simulink model "Linear_Model"  (R2018a)
settings: Solver=VariableStepAuto  StartTime=0.0  StopTime=300  RelTol=1e-3
values from neighbouring files (symbols this model uses):
  A_lat = [a11_lat, a12_lat, a13_lat, a14_lat, a15_lat ... (first row only)    [cont_code-1.m]    (also in flight_controller.m)
  A_long = [a11_long, a12_long, a13_long, a14_long, a15_long ... (first row only)    [cont_code-1.m]    (also in flight_controller.m)
  B_lat = [b11_lat, b12_lat ... (first row only)    [cont_code-1.m]    (also in flight_controller.m)
  B_long = [b11_long, b12_long ... (first row only)    [cont_code-1.m]    (also in flight_controller.m)
  C_lat = eye(5)    [cont_code-1.m]    (also in flight_controller.m)
  C_long = eye(5)    [cont_code-1.m]    (also in flight_controller.m)
  D_lat = zeros(5,2)    [cont_code-1.m]    (also in flight_controller.m)
  D_long = [0, 0 ... (first row only)    [cont_code-1.m]    (also in flight_controller.m)
libraries: simulink x2
settings Model: Creator=Navneet  LastModifiedBy=Sam
settings DebuggingCC: LibraryContextMissingDiagnostic=warning
settings SFSimCC: SimUseLocalCustomCode=on
settings RTWCC: RTWUseLocalCustomCode=on

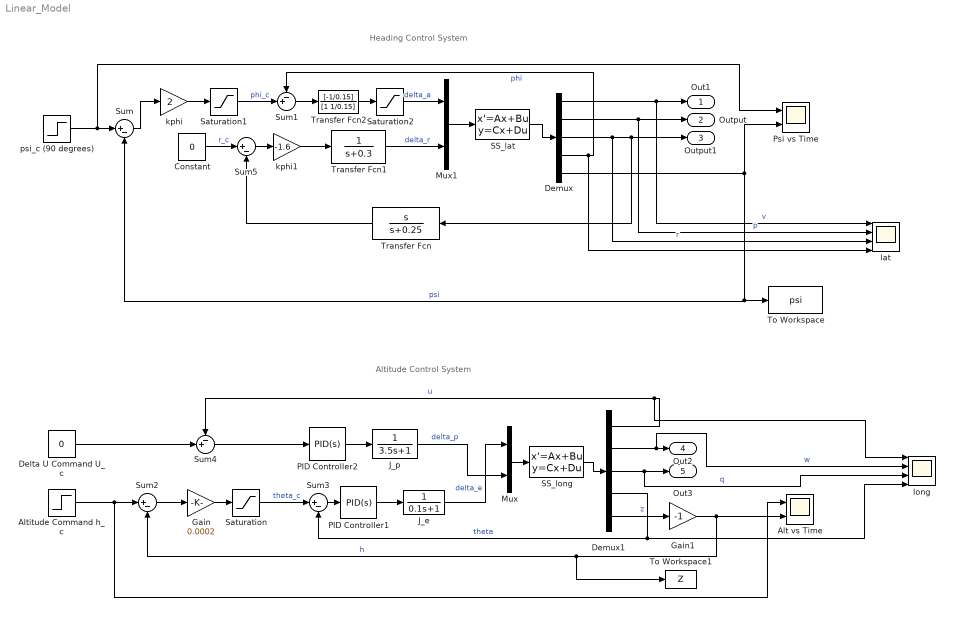
== system Linear_Model ==
  note: Altitude Control System
  note: Heading Control System
  Alt vs Time : Scope  NumInputPorts=2
  Altitude Command h_c : Step  After=1524  SampleTime=0
  Constant : Constant  Value=0
  Delta U Command U_c : Constant  Value=0
  Demux : Demux  Outputs=5
  Demux1 : Demux  Outputs=5
  Gain : Gain  Gain=0.0002
  Gain1 : Gain  Gain=-1
  J_e : TransferFcn  Denominator=[0.1 1]
  J_p : TransferFcn  Denominator=[3.5 1]
  Mux : Mux  Inputs=2
  Mux1 : Mux  Inputs=2
  PID Controller1 : simulink/Continuous/PID Controller  Controller=PID  TimeDomain=Continuous-time  SampleTime=-1  IntegratorMethod=Forward Euler  FilterMethod=Forward Euler  Form=Parallel  UseFilter=on  ControllerParametersSource=internal  P=-6.29147828725261  I=-1.81540038520091  D=-5.41857533868541  N=645.661916939529  InitialConditionSource=internal  InitialConditionForIntegrator=0  InitialConditionForFilter=0  ExternalReset=none  LimitOutput=off  UpperSaturationLimit=inf  LowerSaturationLimit=-inf  LinearizeAsGain=on  AntiWindupMode=none  Kb=1  TrackingMode=off  Kt=1  PParamMin=[]  PParamMax=[]  IParamMin=[]  IParamMax=[]  DParamMin=[]  DParamMax=[]  NParamMin=[]  NParamMax=[]  KbParamMin=[]  KbParamMax=[]  KtParamMin=[]  KtParamMax=[]  POutMin=[]  POutMax=[]  IOutMin=[]  IOutMax=[]  DOutMin=[]  DOutMax=[]  NOutMin=[]  NOutMax=[]  KbOutMin=[]  KbOutMax=[]  KtOutMin=[]  KtOutMax=[]  IntegratorOutMin=[]  IntegratorOutMax=[]  FilterOutMin=[]  FilterOutMax=[]  SumOutMin=[]  SumOutMax=[]  SumI1OutMin=[]  SumI1OutMax=[]  SumI2OutMin=[]  SumI2OutMax=[]  SumI3OutMin=[]  SumI3OutMax=[]  SumDOutMin=[]  SumDOutMax=[]  SaturationOutMin=[]  SaturationOutMax=[]  IntegratorContinuousStateAttributes=''  IntegratorStateMustResolveToSignalObject=off  IntegratorRTWStateStorageClass=Auto  FilterContinuousStateAttributes=''  FilterStateMustResolveToSignalObject=off  FilterRTWStateStorageClass=Auto  DifferentiatorICPrevScaledInput=0  DifferentiatorOutMin=[]  DifferentiatorOutMax=[]  FilterDiffOutCoefMin=[]  FilterDiffOutCoefMax=[]  SumDenOutMin=[]  SumDenOutMax=[]  SumNumOutMin=[]  SumNumOutMax=[]  ReciprocalOutMin=[]  ReciprocalOutMax=[]  DivideOutMin=[]  DivideOutMax=[]  TunerSelectOption=Transfer Function Based (PID Tuner App)
  PID Controller2 : simulink/Continuous/PID Controller  Controller=PID  TimeDomain=Continuous-time  SampleTime=-1  IntegratorMethod=Forward Euler  FilterMethod=Forward Euler  Form=Parallel  UseFilter=on  ControllerParametersSource=internal  P=23.4112253132064  I=10.8898679236466  D=12.4928821977603  N=1211.32658735594  InitialConditionSource=internal  InitialConditionForIntegrator=0  InitialConditionForFilter=0  ExternalReset=none  LimitOutput=off  UpperSaturationLimit=inf  LowerSaturationLimit=-inf  LinearizeAsGain=on  AntiWindupMode=none  Kb=1  TrackingMode=off  Kt=1  PParamMin=[]  PParamMax=[]  IParamMin=[]  IParamMax=[]  DParamMin=[]  DParamMax=[]  NParamMin=[]  NParamMax=[]  KbParamMin=[]  KbParamMax=[]  KtParamMin=[]  KtParamMax=[]  POutMin=[]  POutMax=[]  IOutMin=[]  IOutMax=[]  DOutMin=[]  DOutMax=[]  NOutMin=[]  NOutMax=[]  KbOutMin=[]  KbOutMax=[]  KtOutMin=[]  KtOutMax=[]  IntegratorOutMin=[]  IntegratorOutMax=[]  FilterOutMin=[]  FilterOutMax=[]  SumOutMin=[]  SumOutMax=[]  SumI1OutMin=[]  SumI1OutMax=[]  SumI2OutMin=[]  SumI2OutMax=[]  SumI3OutMin=[]  SumI3OutMax=[]  SumDOutMin=[]  SumDOutMax=[]  SaturationOutMin=[]  SaturationOutMax=[]  IntegratorContinuousStateAttributes=''  IntegratorStateMustResolveToSignalObject=off  IntegratorRTWStateStorageClass=Auto  FilterContinuousStateAttributes=''  FilterStateMustResolveToSignalObject=off  FilterRTWStateStorageClass=Auto  DifferentiatorICPrevScaledInput=0  DifferentiatorOutMin=[]  DifferentiatorOutMax=[]  FilterDiffOutCoefMin=[]  FilterDiffOutCoefMax=[]  SumDenOutMin=[]  SumDenOutMax=[]  SumNumOutMin=[]  SumNumOutMax=[]  ReciprocalOutMin=[]  ReciprocalOutMax=[]  DivideOutMin=[]  DivideOutMax=[]  TunerSelectOption=Transfer Function Based (PID Tuner App)
  Psi vs Time : Scope  NumInputPorts=2
  SS_lat : StateSpace  A=A_lat  B=B_lat  C=C_lat  D=D_lat  InitialCondition=0  ContinuousStateAttributes={'v','p','r','phi','psi'}
  SS_long : StateSpace  A=A_long  B=B_long  C=C_long  D=D_long  InitialCondition=0  ContinuousStateAttributes={'u','w','q','theta','Z'}
  Saturation : Saturate  UpperLimit=5*3.14159/180  LowerLimit=-20*3.14159/180
  Saturation1 : Saturate  UpperLimit=35*3.14/180  LowerLimit=-35*3.14/180
  Saturation2 : Saturate  UpperLimit=10*3.14/180  LowerLimit=-10*3.14/180
  Sum{,2..3,5} (4 alike) : Sum  Inputs=|+-
  Sum1 : Sum  Inputs=-+|
  Sum4 : Sum  Inputs=-+|
  To Workspace : ToWorkspace  VariableName=psi  SampleTime=-1
  To Workspace1 : ToWorkspace  VariableName=Z  SampleTime=-1
  Transfer Fcn : TransferFcn  Numerator=[1 0]  Denominator=[1 0.25]
  Transfer Fcn1 : TransferFcn  Denominator=[1 0.3]
  Transfer Fcn2 : TransferFcn  Numerator=[-1/0.15]  Denominator=[1 1/0.15]
  kphi : Gain  Gain=2
  kphi1 : Gain  Gain=-1.6
  lat : Scope  NumInputPorts=4
  long : Scope  NumInputPorts=4
  psi_c (90 degrees) : Step  After=3.14/2  SampleTime=0
  Out1 : Outport
  Output : Outport  Port=2
  Output1 : Outport  Port=3
  Out2 : Outport  Port=4
  Out3 : Outport  Port=5
  wires:
  Transfer Fcn2/1 -> Saturation2/1
  Sum1/1 -> Transfer Fcn2/1
  Saturation2/1 -> Mux1/1  "delta_a"
  kphi/1 -> Saturation1/1
  Demux/2 -> lat/2, Output/1  "p"
  Demux/3 -> lat/3, Transfer Fcn/1, Output1/1  "r"
  psi_c (90 degrees)/1 -> Sum/1, Psi vs Time/1
  Demux/1 -> lat/1, Out1/1  "v"
  Mux1/1 -> SS_lat/1
  Demux/5 -> Psi vs Time/2, To Workspace/1, Sum/2  "psi"
  Sum/1 -> kphi/1
  SS_lat/1 -> Demux/1
  PID Controller1/1 -> J_e/1
  Altitude Command h_c/1 -> Sum2/1, Alt vs Time/1
  J_e/1 -> Mux/1  "delta_e"
  SS_long/1 -> Demux1/1
  Mux/1 -> SS_long/1
  Gain/1 -> Saturation/1
  Gain1/1 -> To Workspace1/1, Sum2/2, Alt vs Time/2  "h"
  PID Controller2/1 -> J_p/1
  Sum4/1 -> PID Controller2/1
  Demux1/1 -> long/1, Sum4/1  "u"
  Demux1/4 -> Sum3/2, long/4  "theta"
  Demux1/5 -> Gain1/1  "z"
  Delta U Command U_c/1 -> Sum4/2
  Sum3/1 -> PID Controller1/1
  Saturation/1 -> Sum3/1  "theta_c"
  Sum2/1 -> Gain/1
  J_p/1 -> Mux/2  "delta_p"
  Demux1/2 -> long/2, Out2/1  "w"
  Demux1/3 -> long/3, Out3/1  "q"
  Demux/4 -> lat/4, Sum1/1  "phi"
  Saturation1/1 -> Sum1/2  "phi_c"
  Constant/1 -> Sum5/1  "r_c"
  Transfer Fcn/1 -> Sum5/2
  Sum5/1 -> kphi1/1
  Transfer Fcn1/1 -> Mux1/2  "delta_r"
  kphi1/1 -> Transfer Fcn1/1
